simulink model "Observador_estados_discreto_plantilla"  (R2016a)
settings: Solver=VariableStepAuto  StartTime=0.0  StopTime=30  RelTol=1e-3
values from neighbouring files (symbols this model uses):
  A = [-1,0;0,2]    [Regulador_seguidor_observador_codigo.m]
  B = [1;1]    [Regulador_seguidor_observador_codigo.m]
  C = [1,1]    [Regulador_seguidor_observador_codigo.m]
  h = place(A_dis',C_dis',Po)'    [Regulador_seguidor_observador_codigo.m]
  ki = k(1:1,3:3)    [Regulador_seguidor_observador_codigo.m]
  kp = k(1:1,1:2)    [Regulador_seguidor_observador_codigo.m]
  tm = 0.1    [Regulador_seguidor_observador_codigo.m]
undefined symbols (not defined in the file or in its folder): A_dis, B_dis, C_dis
settings Model: Creator=Daniel  LastModifiedBy=Daniel

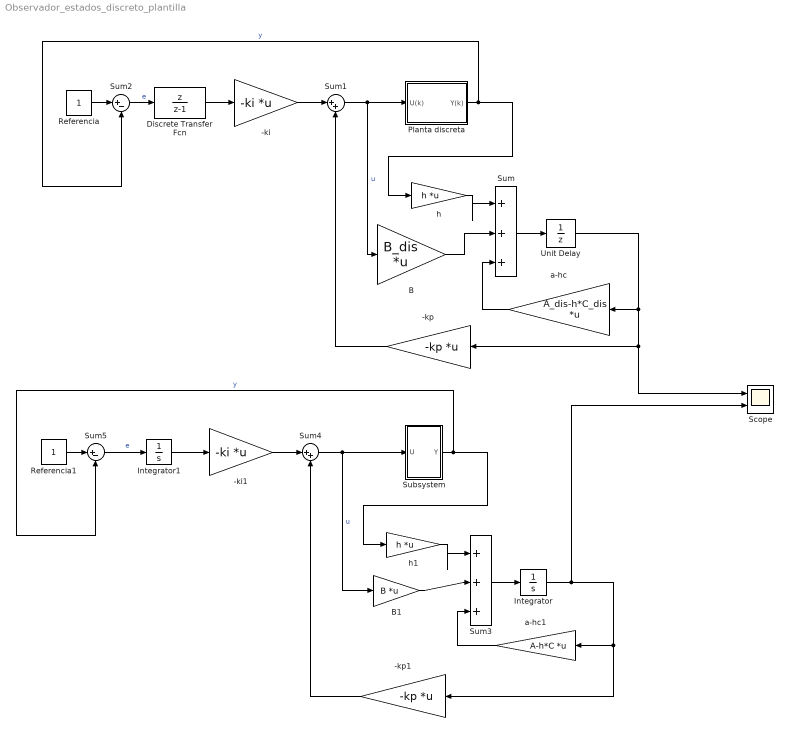
== system Observador_estados_discreto_plantilla ==
  -ki : Gain  Gain=-ki  Multiplication=Matrix(K*u) (u vector)
  -ki1 : Gain  Gain=-ki  Multiplication=Matrix(K*u) (u vector)
  -kp : Gain  Gain=-kp  Multiplication=Matrix(K*u) (u vector)
  -kp1 : Gain  Gain=-kp  Multiplication=Matrix(K*u) (u vector)
  B : Gain  Gain=B_dis  Multiplication=Matrix(K*u) (u vector)
  B1 : Gain  Gain=B  Multiplication=Matrix(K*u) (u vector)
  Discrete Transfer Fcn : DiscreteTransferFcn  Numerator=[1 0]  Denominator=[1 -1]  SampleTime=tm
  Integrator : Integrator
  Integrator1 : Integrator
  Planta discreta : Subsystem
  Referencia : Constant
  Referencia1 : Constant
  Scope : Scope  NumInputPorts=2
  Subsystem : Subsystem
  Sum : Sum  Inputs=|+++
  Sum1 : Sum  Inputs=|++
  Sum2 : Sum  Inputs=|+-
  Sum3 : Sum  Inputs=|+++
  Sum4 : Sum  Inputs=|++
  Sum5 : Sum  Inputs=|+-
  Unit Delay : UnitDelay  SampleTime=tm
  a-hc : Gain  Gain=A_dis-h*C_dis  Multiplication=Matrix(K*u) (u vector)
  a-hc1 : Gain  Gain=A-h*C  Multiplication=Matrix(K*u) (u vector)
  h : Gain  Gain=h  Multiplication=Matrix(K*u) (u vector)
  h1 : Gain  Gain=h  Multiplication=Matrix(K*u) (u vector)
  wires:
  Sum/1 -> Unit Delay/1
  a-hc/1 -> Sum/3
  B/1 -> Sum/2
  h/1 -> Sum/1
  Planta discreta/1(Y(k)) -> Sum2/2, h/1  "y"
  Sum1/1 -> Planta discreta/1(U(k)), B/1  "u"
  Discrete Transfer Fcn/1 -> -ki/1
  Sum2/1 -> Discrete Transfer Fcn/1  "e"
  Referencia/1 -> Sum2/1
  -ki/1 -> Sum1/1
  -kp/1 -> Sum1/2
  Sum3/1 -> Integrator/1
  a-hc1/1 -> Sum3/3
  B1/1 -> Sum3/2
  h1/1 -> Sum3/1
  Subsystem/1(Y) -> h1/1, Sum5/2  "y"
  Sum4/1 -> Subsystem/1(U), B1/1  "u"
  Integrator1/1 -> -ki1/1
  Sum5/1 -> Integrator1/1  "e"
  Referencia1/1 -> Sum5/1
  -ki1/1 -> Sum4/1
  -kp1/1 -> Sum4/2
  Unit Delay/1 -> Scope/1, -kp/1, a-hc/1
  Integrator/1 -> Scope/2, -kp1/1, a-hc1/1

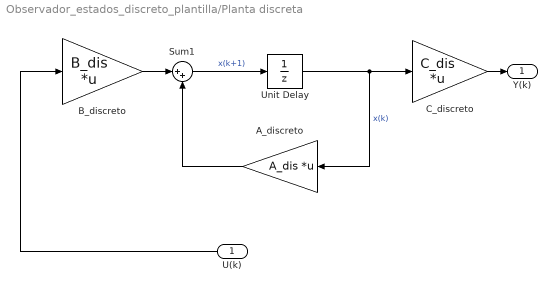
== system Observador_estados_discreto_plantilla/Planta discreta ==
  U(k) : Inport
  A_discreto : Gain  Gain=A_dis  Multiplication=Matrix(K*u) (u vector)
  B_discreto : Gain  Gain=B_dis  Multiplication=Matrix(K*u) (u vector)
  C_discreto : Gain  Gain=C_dis  Multiplication=Matrix(K*u) (u vector)
  Sum1 : Sum  Inputs=|++
  Unit Delay : UnitDelay  SampleTime=tm
  Y(k) : Outport
  wires:
  Unit Delay/1 -> A_discreto/1, C_discreto/1  "x(k)"
  A_discreto/1 -> Sum1/2
  Sum1/1 -> Unit Delay/1  "x(k+1)"
  C_discreto/1 -> Y(k)/1
  U(k)/1 -> B_discreto/1
  B_discreto/1 -> Sum1/1

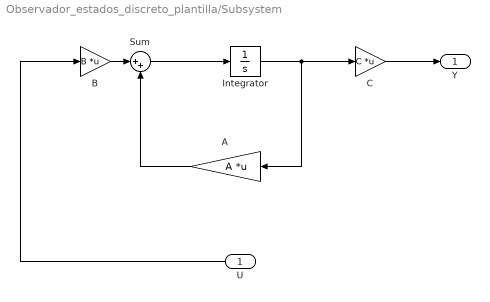
== system Observador_estados_discreto_plantilla/Subsystem ==
  U : Inport
  A : Gain  Gain=A  Multiplication=Matrix(K*u) (u vector)
  B : Gain  Gain=B  Multiplication=Matrix(K*u) (u vector)
  C : Gain  Gain=C  Multiplication=Matrix(K*u) (u vector)
  Integrator : Integrator
  Sum : Sum  Inputs=|++
  Y : Outport
  wires:
  Sum/1 -> Integrator/1
  A/1 -> Sum/2
  U/1 -> B/1
  B/1 -> Sum/1
  C/1 -> Y/1
  Integrator/1 -> A/1, C/1
